simulink model "FaceDet_x4"  (Simulink 7.7)
settings: Solver=FixedStepDiscrete  StartTime=0  StopTime=10  RelTol=1e-3
libraries: simulink x257
(part 3 of 5)

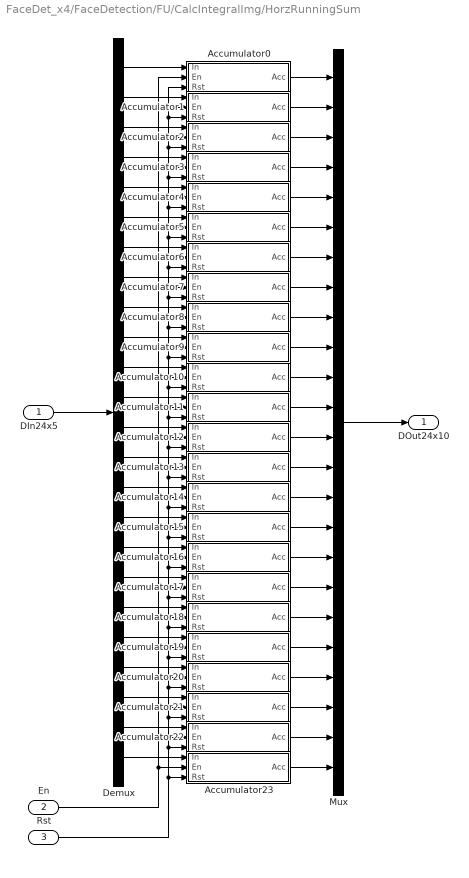
== system FaceDet_x4/FaceDetection/FU/CalcIntegralImg/HorzRunningSum ==
  DIn24x5 : Inport
  En : Inport  Port=2
  Rst : Inport  Port=3
  Accumulator0 : Subsystem  TreatAsAtomicUnit=on  mask(Accumulator){NBits=10}
      mask prompts: NBits "Number of Bits"
      mask help:
      | Accumulates incoming data. On reset only the state is initialized, meaning that when the reset is asserted the first valid output will be available from the next clock.
      | It is user responsiblity not to overcome the capacity of the accumulator.
      mask Help: web( ['E:\Ilia\Sightic\MakeVerilog\AccBlk\', 'AccBlkHelp.htm'] )
      mask Display: disp( 'Acc Blk\nBDelay = 0' )
  Accumulator1 : Subsystem  TreatAsAtomicUnit=on  mask(Accumulator){NBits=10}
      mask prompts: NBits "Number of Bits"
      mask help:
      | Accumulates incoming data. On reset only the state is initialized, meaning that when the reset is asserted the first valid output will be available from the next clock.
      | It is user responsiblity not to overcome the capacity of the accumulator.
      mask Help: web( ['E:\Ilia\Sightic\MakeVerilog\AccBlk\', 'AccBlkHelp.htm'] )
      mask Display: disp( 'Acc Blk\nBDelay = 0' )
  Accumulator10 : Subsystem  TreatAsAtomicUnit=on  mask(Accumulator){NBits=10}
      mask prompts: NBits "Number of Bits"
      mask help:
      | Accumulates incoming data. On reset only the state is initialized, meaning that when the reset is asserted the first valid output will be available from the next clock.
      | It is user responsiblity not to overcome the capacity of the accumulator.
      mask Help: web( ['E:\Ilia\Sightic\MakeVerilog\AccBlk\', 'AccBlkHelp.htm'] )
      mask Display: disp( 'Acc Blk\nBDelay = 0' )
  Accumulator11 : Subsystem  TreatAsAtomicUnit=on  mask(Accumulator){NBits=10}
      mask prompts: NBits "Number of Bits"
      mask help:
      | Accumulates incoming data. On reset only the state is initialized, meaning that when the reset is asserted the first valid output will be available from the next clock.
      | It is user responsiblity not to overcome the capacity of the accumulator.
      mask Help: web( ['E:\Ilia\Sightic\MakeVerilog\AccBlk\', 'AccBlkHelp.htm'] )
      mask Display: disp( 'Acc Blk\nBDelay = 0' )
  Accumulator12 : Subsystem  TreatAsAtomicUnit=on  mask(Accumulator){NBits=10}
      mask prompts: NBits "Number of Bits"
      mask help:
      | Accumulates incoming data. On reset only the state is initialized, meaning that when the reset is asserted the first valid output will be available from the next clock.
      | It is user responsiblity not to overcome the capacity of the accumulator.
      mask Help: web( ['E:\Ilia\Sightic\MakeVerilog\AccBlk\', 'AccBlkHelp.htm'] )
      mask Display: disp( 'Acc Blk\nBDelay = 0' )
  Accumulator13 : Subsystem  TreatAsAtomicUnit=on  mask(Accumulator){NBits=10}
      mask prompts: NBits "Number of Bits"
      mask help:
      | Accumulates incoming data. On reset only the state is initialized, meaning that when the reset is asserted the first valid output will be available from the next clock.
      | It is user responsiblity not to overcome the capacity of the accumulator.
      mask Help: web( ['E:\Ilia\Sightic\MakeVerilog\AccBlk\', 'AccBlkHelp.htm'] )
      mask Display: disp( 'Acc Blk\nBDelay = 0' )
  Accumulator14 : Subsystem  TreatAsAtomicUnit=on  mask(Accumulator){NBits=10}
      mask prompts: NBits "Number of Bits"
      mask help:
      | Accumulates incoming data. On reset only the state is initialized, meaning that when the reset is asserted the first valid output will be available from the next clock.
      | It is user responsiblity not to overcome the capacity of the accumulator.
      mask Help: web( ['E:\Ilia\Sightic\MakeVerilog\AccBlk\', 'AccBlkHelp.htm'] )
      mask Display: disp( 'Acc Blk\nBDelay = 0' )
  Accumulator15 : Subsystem  TreatAsAtomicUnit=on  mask(Accumulator){NBits=10}
      mask prompts: NBits "Number of Bits"
      mask help:
      | Accumulates incoming data. On reset only the state is initialized, meaning that when the reset is asserted the first valid output will be available from the next clock.
      | It is user responsiblity not to overcome the capacity of the accumulator.
      mask Help: web( ['E:\Ilia\Sightic\MakeVerilog\AccBlk\', 'AccBlkHelp.htm'] )
      mask Display: disp( 'Acc Blk\nBDelay = 0' )
  Accumulator16 : Subsystem  TreatAsAtomicUnit=on  mask(Accumulator){NBits=10}
      mask prompts: NBits "Number of Bits"
      mask help:
      | Accumulates incoming data. On reset only the state is initialized, meaning that when the reset is asserted the first valid output will be available from the next clock.
      | It is user responsiblity not to overcome the capacity of the accumulator.
      mask Help: web( ['E:\Ilia\Sightic\MakeVerilog\AccBlk\', 'AccBlkHelp.htm'] )
      mask Display: disp( 'Acc Blk\nBDelay = 0' )
  Accumulator17 : Subsystem  TreatAsAtomicUnit=on  mask(Accumulator){NBits=10}
      mask prompts: NBits "Number of Bits"
      mask help:
      | Accumulates incoming data. On reset only the state is initialized, meaning that when the reset is asserted the first valid output will be available from the next clock.
      | It is user responsiblity not to overcome the capacity of the accumulator.
      mask Help: web( ['E:\Ilia\Sightic\MakeVerilog\AccBlk\', 'AccBlkHelp.htm'] )
      mask Display: disp( 'Acc Blk\nBDelay = 0' )
  Accumulator18 : Subsystem  TreatAsAtomicUnit=on  mask(Accumulator){NBits=10}
      mask prompts: NBits "Number of Bits"
      mask help:
      | Accumulates incoming data. On reset only the state is initialized, meaning that when the reset is asserted the first valid output will be available from the next clock.
      | It is user responsiblity not to overcome the capacity of the accumulator.
      mask Help: web( ['E:\Ilia\Sightic\MakeVerilog\AccBlk\', 'AccBlkHelp.htm'] )
      mask Display: disp( 'Acc Blk\nBDelay = 0' )
  Accumulator19 : Subsystem  TreatAsAtomicUnit=on  mask(Accumulator){NBits=10}
      mask prompts: NBits "Number of Bits"
      mask help:
      | Accumulates incoming data. On reset only the state is initialized, meaning that when the reset is asserted the first valid output will be available from the next clock.
      | It is user responsiblity not to overcome the capacity of the accumulator.
      mask Help: web( ['E:\Ilia\Sightic\MakeVerilog\AccBlk\', 'AccBlkHelp.htm'] )
      mask Display: disp( 'Acc Blk\nBDelay = 0' )
  Accumulator2 : Subsystem  TreatAsAtomicUnit=on  mask(Accumulator){NBits=10}
      mask prompts: NBits "Number of Bits"
      mask help:
      | Accumulates incoming data. On reset only the state is initialized, meaning that when the reset is asserted the first valid output will be available from the next clock.
      | It is user responsiblity not to overcome the capacity of the accumulator.
      mask Help: web( ['E:\Ilia\Sightic\MakeVerilog\AccBlk\', 'AccBlkHelp.htm'] )
      mask Display: disp( 'Acc Blk\nBDelay = 0' )
  Accumulator20 : Subsystem  TreatAsAtomicUnit=on  mask(Accumulator){NBits=10}
      mask prompts: NBits "Number of Bits"
      mask help:
      | Accumulates incoming data. On reset only the state is initialized, meaning that when the reset is asserted the first valid output will be available from the next clock.
      | It is user responsiblity not to overcome the capacity of the accumulator.
      mask Help: web( ['E:\Ilia\Sightic\MakeVerilog\AccBlk\', 'AccBlkHelp.htm'] )
      mask Display: disp( 'Acc Blk\nBDelay = 0' )
  Accumulator21 : Subsystem  TreatAsAtomicUnit=on  mask(Accumulator){NBits=10}
      mask prompts: NBits "Number of Bits"
      mask help:
      | Accumulates incoming data. On reset only the state is initialized, meaning that when the reset is asserted the first valid output will be available from the next clock.
      | It is user responsiblity not to overcome the capacity of the accumulator.
      mask Help: web( ['E:\Ilia\Sightic\MakeVerilog\AccBlk\', 'AccBlkHelp.htm'] )
      mask Display: disp( 'Acc Blk\nBDelay = 0' )
  Accumulator22 : Subsystem  TreatAsAtomicUnit=on  mask(Accumulator){NBits=10}
      mask prompts: NBits "Number of Bits"
      mask help:
      | Accumulates incoming data. On reset only the state is initialized, meaning that when the reset is asserted the first valid output will be available from the next clock.
      | It is user responsiblity not to overcome the capacity of the accumulator.
      mask Help: web( ['E:\Ilia\Sightic\MakeVerilog\AccBlk\', 'AccBlkHelp.htm'] )
      mask Display: disp( 'Acc Blk\nBDelay = 0' )
  Accumulator23 : Subsystem  TreatAsAtomicUnit=on  mask(Accumulator){NBits=10}
      mask prompts: NBits "Number of Bits"
      mask help:
      | Accumulates incoming data. On reset only the state is initialized, meaning that when the reset is asserted the first valid output will be available from the next clock.
      | It is user responsiblity not to overcome the capacity of the accumulator.
      mask Help: web( ['E:\Ilia\Sightic\MakeVerilog\AccBlk\', 'AccBlkHelp.htm'] )
      mask Display: disp( 'Acc Blk\nBDelay = 0' )
  Accumulator3 : Subsystem  TreatAsAtomicUnit=on  mask(Accumulator){NBits=10}
      mask prompts: NBits "Number of Bits"
      mask help:
      | Accumulates incoming data. On reset only the state is initialized, meaning that when the reset is asserted the first valid output will be available from the next clock.
      | It is user responsiblity not to overcome the capacity of the accumulator.
      mask Help: web( ['E:\Ilia\Sightic\MakeVerilog\AccBlk\', 'AccBlkHelp.htm'] )
      mask Display: disp( 'Acc Blk\nBDelay = 0' )
  Accumulator4 : Subsystem  TreatAsAtomicUnit=on  mask(Accumulator){NBits=10}
      mask prompts: NBits "Number of Bits"
      mask help:
      | Accumulates incoming data. On reset only the state is initialized, meaning that when the reset is asserted the first valid output will be available from the next clock.
      | It is user responsiblity not to overcome the capacity of the accumulator.
      mask Help: web( ['E:\Ilia\Sightic\MakeVerilog\AccBlk\', 'AccBlkHelp.htm'] )
      mask Display: disp( 'Acc Blk\nBDelay = 0' )
  Accumulator5 : Subsystem  TreatAsAtomicUnit=on  mask(Accumulator){NBits=10}
      mask prompts: NBits "Number of Bits"
      mask help:
      | Accumulates incoming data. On reset only the state is initialized, meaning that when the reset is asserted the first valid output will be available from the next clock.
      | It is user responsiblity not to overcome the capacity of the accumulator.
      mask Help: web( ['E:\Ilia\Sightic\MakeVerilog\AccBlk\', 'AccBlkHelp.htm'] )
      mask Display: disp( 'Acc Blk\nBDelay = 0' )
  Accumulator6 : Subsystem  TreatAsAtomicUnit=on  mask(Accumulator){NBits=10}
      mask prompts: NBits "Number of Bits"
      mask help:
      | Accumulates incoming data. On reset only the state is initialized, meaning that when the reset is asserted the first valid output will be available from the next clock.
      | It is user responsiblity not to overcome the capacity of the accumulator.
      mask Help: web( ['E:\Ilia\Sightic\MakeVerilog\AccBlk\', 'AccBlkHelp.htm'] )
      mask Display: disp( 'Acc Blk\nBDelay = 0' )
  Accumulator7 : Subsystem  TreatAsAtomicUnit=on  mask(Accumulator){NBits=10}
      mask prompts: NBits "Number of Bits"
      mask help:
      | Accumulates incoming data. On reset only the state is initialized, meaning that when the reset is asserted the first valid output will be available from the next clock.
      | It is user responsiblity not to overcome the capacity of the accumulator.
      mask Help: web( ['E:\Ilia\Sightic\MakeVerilog\AccBlk\', 'AccBlkHelp.htm'] )
      mask Display: disp( 'Acc Blk\nBDelay = 0' )
  Accumulator8 : Subsystem  TreatAsAtomicUnit=on  mask(Accumulator){NBits=10}
      mask prompts: NBits "Number of Bits"
      mask help:
      | Accumulates incoming data. On reset only the state is initialized, meaning that when the reset is asserted the first valid output will be available from the next clock.
      | It is user responsiblity not to overcome the capacity of the accumulator.
      mask Help: web( ['E:\Ilia\Sightic\MakeVerilog\AccBlk\', 'AccBlkHelp.htm'] )
      mask Display: disp( 'Acc Blk\nBDelay = 0' )
  Accumulator9 : Subsystem  TreatAsAtomicUnit=on  mask(Accumulator){NBits=10}
      mask prompts: NBits "Number of Bits"
      mask help:
      | Accumulates incoming data. On reset only the state is initialized, meaning that when the reset is asserted the first valid output will be available from the next clock.
      | It is user responsiblity not to overcome the capacity of the accumulator.
      mask Help: web( ['E:\Ilia\Sightic\MakeVerilog\AccBlk\', 'AccBlkHelp.htm'] )
      mask Display: disp( 'Acc Blk\nBDelay = 0' )
  Demux : Demux  Outputs=24
  Mux : Mux  Inputs=24
  DOut24x10 : Outport  RequirementInfo={} %GIDa_f25d4dfd_08ec_4fe4_83ec_06833589800f
  wires:
  DIn24x5/1 -> Demux/1
  Mux/1 -> DOut24x10/1
  Demux/1 -> Accumulator0/1(In)
  Demux/2 -> Accumulator1/1(In)
  Demux/3 -> Accumulator2/1(In)
  Demux/4 -> Accumulator3/1(In)
  Demux/5 -> Accumulator4/1(In)
  Demux/6 -> Accumulator5/1(In)
  Demux/7 -> Accumulator6/1(In)
  Demux/8 -> Accumulator7/1(In)
  Demux/9 -> Accumulator8/1(In)
  Demux/10 -> Accumulator9/1(In)
  Demux/11 -> Accumulator10/1(In)
  Demux/12 -> Accumulator11/1(In)
  Demux/13 -> Accumulator12/1(In)
  Demux/14 -> Accumulator13/1(In)
  Demux/15 -> Accumulator14/1(In)
  Demux/16 -> Accumulator15/1(In)
  Demux/17 -> Accumulator16/1(In)
  Demux/18 -> Accumulator17/1(In)
  Demux/19 -> Accumulator18/1(In)
  Demux/20 -> Accumulator19/1(In)
  Demux/21 -> Accumulator20/1(In)
  Demux/22 -> Accumulator21/1(In)
  Demux/23 -> Accumulator22/1(In)
  Demux/24 -> Accumulator23/1(In)
  En/1 -> Accumulator0/2(En), Accumulator1/2(En), Accumulator2/2(En), Accumulator3/2(En), Accumulator4/2(En), Accumulator5/2(En), Accumulator6/2(En), Accumulator7/2(En), Accumulator8/2(En), Accumulator9/2(En), Accumulator10/2(En), Accumulator11/2(En), Accumulator12/2(En), Accumulator13/2(En), Accumulator14/2(En), Accumulator15/2(En), Accumulator16/2(En), Accumulator17/2(En), Accumulator18/2(En), Accumulator19/2(En), Accumulator20/2(En), Accumulator21/2(En), Accumulator22/2(En), Accumulator23/2(En)
  Rst/1 -> Accumulator0/3(Rst), Accumulator1/3(Rst), Accumulator2/3(Rst), Accumulator3/3(Rst), Accumulator4/3(Rst), Accumulator5/3(Rst), Accumulator6/3(Rst), Accumulator7/3(Rst), Accumulator8/3(Rst), Accumulator9/3(Rst), Accumulator10/3(Rst), Accumulator11/3(Rst), Accumulator12/3(Rst), Accumulator13/3(Rst), Accumulator14/3(Rst), Accumulator15/3(Rst), Accumulator16/3(Rst), Accumulator17/3(Rst), Accumulator18/3(Rst), Accumulator19/3(Rst), Accumulator20/3(Rst), Accumulator21/3(Rst), Accumulator22/3(Rst), Accumulator23/3(Rst)
  Accumulator0/1(Acc) -> Mux/1
  Accumulator1/1(Acc) -> Mux/2
  Accumulator2/1(Acc) -> Mux/3
  Accumulator3/1(Acc) -> Mux/4
  Accumulator4/1(Acc) -> Mux/5
  Accumulator5/1(Acc) -> Mux/6
  Accumulator6/1(Acc) -> Mux/7
  Accumulator7/1(Acc) -> Mux/8
  Accumulator8/1(Acc) -> Mux/9
  Accumulator9/1(Acc) -> Mux/10
  Accumulator10/1(Acc) -> Mux/11
  Accumulator11/1(Acc) -> Mux/12
  Accumulator12/1(Acc) -> Mux/13
  Accumulator13/1(Acc) -> Mux/14
  Accumulator14/1(Acc) -> Mux/15
  Accumulator15/1(Acc) -> Mux/16
  Accumulator16/1(Acc) -> Mux/17
  Accumulator17/1(Acc) -> Mux/18
  Accumulator18/1(Acc) -> Mux/19
  Accumulator19/1(Acc) -> Mux/20
  Accumulator20/1(Acc) -> Mux/21
  Accumulator21/1(Acc) -> Mux/22
  Accumulator22/1(Acc) -> Mux/23
  Accumulator23/1(Acc) -> Mux/24

== system FaceDet_x4/FaceDetection/FU/CalcIntegralImg/TestValidNN ==
  MeanBlkVal : Inport
  Logical Operator : Logic  Operator=OR  AllPortsSameDT=off  OutDataTypeStr=boolean
  MeanMax : Constant  Value=17508  OutDataTypeStr=ufix(15)
  MeanMin : Constant  Value=1543  OutDataTypeStr=ufix(11)
  PassFail : Logic  Operator=NOT  AllPortsSameDT=off  OutDataTypeStr=boolean
  UnitDelay : UnitDelay
  aboveMax : RelationalOperator  Operator=>  OutDataTypeStr=boolean
  belowMin : RelationalOperator  Operator=<  OutDataTypeStr=boolean
  ValidNN : Outport
  wires:
  MeanMin/1 -> belowMin/2
  MeanBlkVal/1 -> belowMin/1, aboveMax/1
  aboveMax/1 -> Logical Operator/1
  belowMin/1 -> Logical Operator/2
  Logical Operator/1 -> PassFail/1
  MeanMax/1 -> aboveMax/2
  PassFail/1 -> UnitDelay/1
  UnitDelay/1 -> ValidNN/1

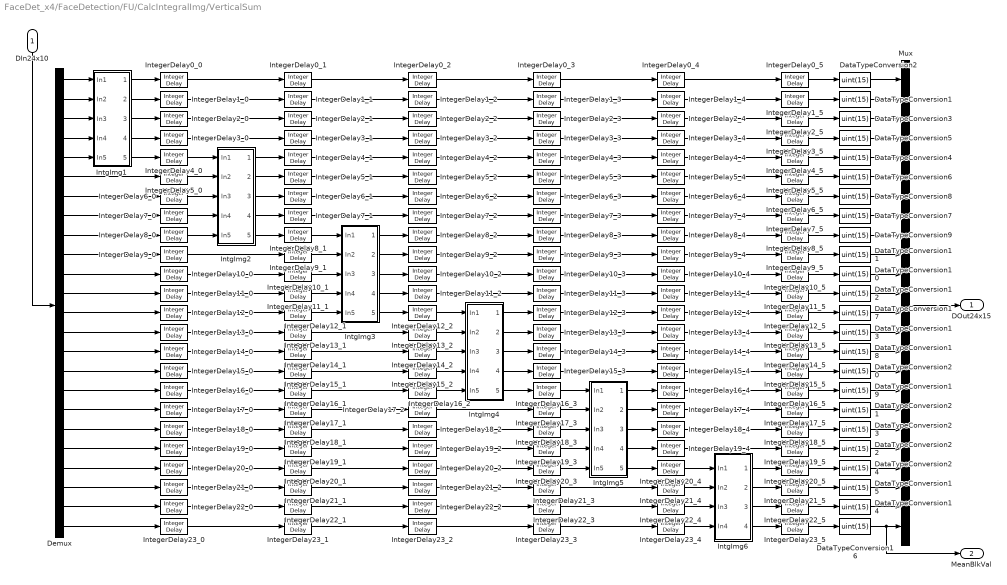
== system FaceDet_x4/FaceDetection/FU/CalcIntegralImg/VerticalSum ==
  DIn24x10 : Inport
  DataTypeConversion{1..24} (24 alike) : DataTypeConversion  OutDataTypeStr=uint(15)
  Demux : Demux  Outputs=24
  IntegerDelay0_{0..5} (6 alike) : simulink/Discrete/Integer Delay  NumDelays=1  InputProcessing=Inherited  vinit=0  samptime=1
  IntegerDelay10_{0..5} (6 alike) : simulink/Discrete/Integer Delay  NumDelays=1  InputProcessing=Inherited  vinit=0  samptime=1
  IntegerDelay11_{0..5} (6 alike) : simulink/Discrete/Integer Delay  NumDelays=1  InputProcessing=Inherited  vinit=0  samptime=1
  IntegerDelay12_{0..5} (6 alike) : simulink/Discrete/Integer Delay  NumDelays=1  InputProcessing=Inherited  vinit=0  samptime=1
  IntegerDelay13_{0..5} (6 alike) : simulink/Discrete/Integer Delay  NumDelays=1  InputProcessing=Inherited  vinit=0  samptime=1
  IntegerDelay14_{0..5} (6 alike) : simulink/Discrete/Integer Delay  NumDelays=1  InputProcessing=Inherited  vinit=0  samptime=1
  IntegerDelay15_{0..5} (6 alike) : simulink/Discrete/Integer Delay  NumDelays=1  InputProcessing=Inherited  vinit=0  samptime=1
  IntegerDelay16_{0..5} (6 alike) : simulink/Discrete/Integer Delay  NumDelays=1  InputProcessing=Inherited  vinit=0  samptime=1
  IntegerDelay17_{0..5} (6 alike) : simulink/Discrete/Integer Delay  NumDelays=1  InputProcessing=Inherited  vinit=0  samptime=1
  IntegerDelay18_{0..5} (6 alike) : simulink/Discrete/Integer Delay  NumDelays=1  InputProcessing=Inherited  vinit=0  samptime=1
  IntegerDelay19_{0..5} (6 alike) : simulink/Discrete/Integer Delay  NumDelays=1  InputProcessing=Inherited  vinit=0  samptime=1
  IntegerDelay1_{0..5} (6 alike) : simulink/Discrete/Integer Delay  NumDelays=1  InputProcessing=Inherited  vinit=0  samptime=1
  IntegerDelay20_{0..5} (6 alike) : simulink/Discrete/Integer Delay  NumDelays=1  InputProcessing=Inherited  vinit=0  samptime=1
  IntegerDelay21_{0..5} (6 alike) : simulink/Discrete/Integer Delay  NumDelays=1  InputProcessing=Inherited  vinit=0  samptime=1
  IntegerDelay22_{0..5} (6 alike) : simulink/Discrete/Integer Delay  NumDelays=1  InputProcessing=Inherited  vinit=0  samptime=1
  IntegerDelay23_{0..5} (6 alike) : simulink/Discrete/Integer Delay  NumDelays=1  InputProcessing=Inherited  vinit=0  samptime=1
  IntegerDelay2_{0..5} (6 alike) : simulink/Discrete/Integer Delay  NumDelays=1  InputProcessing=Inherited  vinit=0  samptime=1
  IntegerDelay3_{0..5} (6 alike) : simulink/Discrete/Integer Delay  NumDelays=1  InputProcessing=Inherited  vinit=0  samptime=1
  IntegerDelay4_{0..5} (6 alike) : simulink/Discrete/Integer Delay  NumDelays=1  InputProcessing=Inherited  vinit=0  samptime=1
  IntegerDelay5_{0..5} (6 alike) : simulink/Discrete/Integer Delay  NumDelays=1  InputProcessing=Inherited  vinit=0  samptime=1
  IntegerDelay6_{0..5} (6 alike) : simulink/Discrete/Integer Delay  NumDelays=1  InputProcessing=Inherited  vinit=0  samptime=1
  IntegerDelay7_{0..5} (6 alike) : simulink/Discrete/Integer Delay  NumDelays=1  InputProcessing=Inherited  vinit=0  samptime=1
  IntegerDelay8_{0..5} (6 alike) : simulink/Discrete/Integer Delay  NumDelays=1  InputProcessing=Inherited  vinit=0  samptime=1
  IntegerDelay9_{0..5} (6 alike) : simulink/Discrete/Integer Delay  NumDelays=1  InputProcessing=Inherited  vinit=0  samptime=1
  IntgImg1 : Subsystem
  IntgImg2 : Subsystem
  IntgImg3 : Subsystem
  IntgImg4 : Subsystem
  IntgImg5 : Subsystem
  IntgImg6 : Subsystem
  Mux : Mux  Inputs=24
  DOut24x15 : Outport
  MeanBlkVal : Outport  Port=2
  wires:
  DIn24x10/1 -> Demux/1
  Demux/1 -> IntgImg1/1(In1)
  Demux/2 -> IntgImg1/2(In2)
  Demux/3 -> IntgImg1/3(In3)
  Demux/6 -> IntegerDelay5_0/1
  IntgImg1/3(Out3) -> IntegerDelay2_0/1
  IntgImg1/1(Out1) -> IntegerDelay0_0/1
  Mux/1 -> DOut24x15/1
  IntgImg1/2(Out2) -> IntegerDelay1_0/1
  IntegerDelay2_0/1 -> IntegerDelay2_1/1
  IntegerDelay3_0/1 -> IntegerDelay3_1/1
  IntegerDelay4_0/1 -> IntgImg2/1(In1)
  Demux/7 -> IntegerDelay6_0/1
  IntegerDelay0_0/1 -> IntegerDelay0_1/1
  Demux/8 -> IntegerDelay7_0/1
  Demux/9 -> IntegerDelay8_0/1
  Demux/10 -> IntegerDelay9_0/1
  Demux/11 -> IntegerDelay10_0/1
  Demux/12 -> IntegerDelay11_0/1
  Demux/13 -> IntegerDelay12_0/1
  Demux/14 -> IntegerDelay13_0/1
  Demux/15 -> IntegerDelay14_0/1
  Demux/16 -> IntegerDelay15_0/1
  Demux/17 -> IntegerDelay16_0/1
  Demux/18 -> IntegerDelay17_0/1
  Demux/19 -> IntegerDelay18_0/1
  Demux/20 -> IntegerDelay19_0/1
  Demux/21 -> IntegerDelay20_0/1
  Demux/22 -> IntegerDelay21_0/1
  Demux/23 -> IntegerDelay22_0/1
  Demux/24 -> IntegerDelay23_0/1
  IntgImg2/1(Out1) -> IntegerDelay4_1/1
  IntegerDelay9_0/1 -> IntegerDelay9_1/1
  IntegerDelay10_0/1 -> IntegerDelay10_1/1
  IntegerDelay11_0/1 -> IntegerDelay11_1/1
  IntegerDelay12_0/1 -> IntegerDelay12_1/1
  IntegerDelay13_0/1 -> IntegerDelay13_1/1
  IntegerDelay14_0/1 -> IntegerDelay14_1/1
  IntegerDelay15_0/1 -> IntegerDelay15_1/1
  IntegerDelay16_0/1 -> IntegerDelay16_1/1
  IntegerDelay17_0/1 -> IntegerDelay17_1/1
  IntegerDelay18_0/1 -> IntegerDelay18_1/1
  IntegerDelay19_0/1 -> IntegerDelay19_1/1
  IntegerDelay20_0/1 -> IntegerDelay20_1/1
  IntegerDelay21_0/1 -> IntegerDelay21_1/1
  IntegerDelay22_0/1 -> IntegerDelay22_1/1
  IntegerDelay23_0/1 -> IntegerDelay23_1/1
  Demux/4 -> IntgImg1/4(In4)
  Demux/5 -> IntgImg1/5(In5)
  IntgImg1/4(Out4) -> IntegerDelay3_0/1
  IntgImg1/5(Out5) -> IntegerDelay4_0/1
  IntegerDelay1_0/1 -> IntegerDelay1_1/1
  IntegerDelay5_0/1 -> IntgImg2/2(In2)
  IntegerDelay6_0/1 -> IntgImg2/3(In3)
  IntegerDelay7_0/1 -> IntgImg2/4(In4)
  IntegerDelay8_0/1 -> IntgImg2/5(In5)
  IntgImg2/2(Out2) -> IntegerDelay5_1/1
  IntgImg2/3(Out3) -> IntegerDelay6_1/1
  IntgImg2/4(Out4) -> IntegerDelay7_1/1
  IntgImg2/5(Out5) -> IntegerDelay8_1/1
  IntegerDelay2_1/1 -> IntegerDelay2_2/1
  IntegerDelay3_1/1 -> IntegerDelay3_2/1
  IntegerDelay0_1/1 -> IntegerDelay0_2/1
  IntegerDelay13_1/1 -> IntegerDelay13_2/1
  IntegerDelay14_1/1 -> IntegerDelay14_2/1
  IntegerDelay15_1/1 -> IntegerDelay15_2/1
  IntegerDelay16_1/1 -> IntegerDelay16_2/1
  IntegerDelay17_1/1 -> IntegerDelay17_2/1
  IntegerDelay18_1/1 -> IntegerDelay18_2/1
  IntegerDelay19_1/1 -> IntegerDelay19_2/1
  IntegerDelay20_1/1 -> IntegerDelay20_2/1
  IntegerDelay21_1/1 -> IntegerDelay21_2/1
  IntegerDelay22_1/1 -> IntegerDelay22_2/1
  IntegerDelay23_1/1 -> IntegerDelay23_2/1
  IntegerDelay1_1/1 -> IntegerDelay1_2/1
  IntegerDelay8_1/1 -> IntgImg3/1(In1)
  IntegerDelay9_1/1 -> IntgImg3/2(In2)
  IntegerDelay10_1/1 -> IntgImg3/3(In3)
  IntegerDelay11_1/1 -> IntgImg3/4(In4)
  IntegerDelay12_1/1 -> IntgImg3/5(In5)
  IntegerDelay4_1/1 -> IntegerDelay4_2/1
  IntegerDelay5_1/1 -> IntegerDelay5_2/1
  IntegerDelay6_1/1 -> IntegerDelay6_2/1
  IntegerDelay7_1/1 -> IntegerDelay7_2/1
  IntgImg3/1(Out1) -> IntegerDelay8_2/1
  IntgImg3/2(Out2) -> IntegerDelay9_2/1
  IntgImg3/3(Out3) -> IntegerDelay10_2/1
  IntgImg3/4(Out4) -> IntegerDelay11_2/1
  IntgImg3/5(Out5) -> IntegerDelay12_2/1
  IntegerDelay2_2/1 -> IntegerDelay2_3/1
  IntegerDelay3_2/1 -> IntegerDelay3_3/1
  IntegerDelay0_2/1 -> IntegerDelay0_3/1
  IntegerDelay17_2/1 -> IntegerDelay17_3/1
  IntegerDelay18_2/1 -> IntegerDelay18_3/1
  IntegerDelay19_2/1 -> IntegerDelay19_3/1
  IntegerDelay20_2/1 -> IntegerDelay20_3/1
  IntegerDelay21_2/1 -> IntegerDelay21_3/1
  IntegerDelay22_2/1 -> IntegerDelay22_3/1
  IntegerDelay23_2/1 -> IntegerDelay23_3/1
  IntegerDelay1_2/1 -> IntegerDelay1_3/1
  IntegerDelay4_2/1 -> IntegerDelay4_3/1
  IntegerDelay5_2/1 -> IntegerDelay5_3/1
  IntegerDelay6_2/1 -> IntegerDelay6_3/1
  IntegerDelay7_2/1 -> IntegerDelay7_3/1
  IntegerDelay8_2/1 -> IntegerDelay8_3/1
  IntegerDelay9_2/1 -> IntegerDelay9_3/1
  IntegerDelay10_2/1 -> IntegerDelay10_3/1
  IntegerDelay11_2/1 -> IntegerDelay11_3/1
  IntegerDelay12_2/1 -> IntgImg4/1(In1)
  IntegerDelay13_2/1 -> IntgImg4/2(In2)
  IntegerDelay14_2/1 -> IntgImg4/3(In3)
  IntegerDelay15_2/1 -> IntgImg4/4(In4)
  IntegerDelay16_2/1 -> IntgImg4/5(In5)
  IntgImg4/1(Out1) -> IntegerDelay12_3/1
  IntgImg4/2(Out2) -> IntegerDelay13_3/1
  IntgImg4/3(Out3) -> IntegerDelay14_3/1
  IntgImg4/4(Out4) -> IntegerDelay15_3/1
  IntgImg4/5(Out5) -> IntegerDelay16_3/1
  IntegerDelay2_3/1 -> IntegerDelay2_4/1
  IntegerDelay3_3/1 -> IntegerDelay3_4/1
  IntegerDelay0_3/1 -> IntegerDelay0_4/1
  IntegerDelay21_3/1 -> IntegerDelay21_4/1
  IntegerDelay22_3/1 -> IntegerDelay22_4/1
  IntegerDelay23_3/1 -> IntegerDelay23_4/1
  IntegerDelay1_3/1 -> IntegerDelay1_4/1
  IntegerDelay4_3/1 -> IntegerDelay4_4/1
  IntegerDelay5_3/1 -> IntegerDelay5_4/1
  IntegerDelay6_3/1 -> IntegerDelay6_4/1
  IntegerDelay7_3/1 -> IntegerDelay7_4/1
  IntegerDelay8_3/1 -> IntegerDelay8_4/1
  IntegerDelay9_3/1 -> IntegerDelay9_4/1
  IntegerDelay10_3/1 -> IntegerDelay10_4/1
  IntegerDelay11_3/1 -> IntegerDelay11_4/1
  IntegerDelay12_3/1 -> IntegerDelay12_4/1
  IntegerDelay13_3/1 -> IntegerDelay13_4/1
  IntegerDelay14_3/1 -> IntegerDelay14_4/1
  IntegerDelay15_3/1 -> IntegerDelay15_4/1
  IntegerDelay16_3/1 -> IntgImg5/1(In1)
  IntegerDelay17_3/1 -> IntgImg5/2(In2)
  IntegerDelay18_3/1 -> IntgImg5/3(In3)
  IntegerDelay19_3/1 -> IntgImg5/4(In4)
  IntegerDelay20_3/1 -> IntgImg5/5(In5)
  IntgImg5/1(Out1) -> IntegerDelay16_4/1
  IntgImg5/2(Out2) -> IntegerDelay17_4/1
  IntgImg5/3(Out3) -> IntegerDelay18_4/1
  IntgImg5/4(Out4) -> IntegerDelay19_4/1
  IntgImg5/5(Out5) -> IntegerDelay20_4/1
  IntegerDelay2_4/1 -> IntegerDelay2_5/1
  IntegerDelay3_4/1 -> IntegerDelay3_5/1
  IntegerDelay0_4/1 -> IntegerDelay0_5/1
  IntegerDelay1_4/1 -> IntegerDelay1_5/1
  IntegerDelay4_4/1 -> IntegerDelay4_5/1
  IntegerDelay5_4/1 -> IntegerDelay5_5/1
  IntegerDelay6_4/1 -> IntegerDelay6_5/1
  IntegerDelay7_4/1 -> IntegerDelay7_5/1
  IntegerDelay8_4/1 -> IntegerDelay8_5/1
  IntegerDelay9_4/1 -> IntegerDelay9_5/1
  IntegerDelay10_4/1 -> IntegerDelay10_5/1
  IntegerDelay11_4/1 -> IntegerDelay11_5/1
  IntegerDelay12_4/1 -> IntegerDelay12_5/1
  IntegerDelay13_4/1 -> IntegerDelay13_5/1
  IntegerDelay14_4/1 -> IntegerDelay14_5/1
  IntegerDelay15_4/1 -> IntegerDelay15_5/1
  IntegerDelay16_4/1 -> IntegerDelay16_5/1
  IntegerDelay17_4/1 -> IntegerDelay17_5/1
  IntegerDelay18_4/1 -> IntegerDelay18_5/1
  IntegerDelay19_4/1 -> IntegerDelay19_5/1
  IntegerDelay20_4/1 -> IntgImg6/1(In1)
  IntegerDelay21_4/1 -> IntgImg6/2(In2)
  IntegerDelay22_4/1 -> IntgImg6/3(In3)
  IntegerDelay23_4/1 -> IntgImg6/4(In4)
  IntgImg6/1(Out1) -> IntegerDelay20_5/1
  IntgImg6/2(Out2) -> IntegerDelay21_5/1
  IntgImg6/3(Out3) -> IntegerDelay22_5/1
  IntgImg6/4(Out4) -> IntegerDelay23_5/1
  IntegerDelay0_5/1 -> DataTypeConversion2/1
  IntegerDelay1_5/1 -> DataTypeConversion1/1
  IntegerDelay2_5/1 -> DataTypeConversion3/1
  IntegerDelay3_5/1 -> DataTypeConversion5/1
  IntegerDelay4_5/1 -> DataTypeConversion4/1
  IntegerDelay5_5/1 -> DataTypeConversion6/1
  IntegerDelay6_5/1 -> DataTypeConversion8/1
  IntegerDelay7_5/1 -> DataTypeConversion7/1
  IntegerDelay8_5/1 -> DataTypeConversion9/1
  IntegerDelay9_5/1 -> DataTypeConversion11/1
  IntegerDelay10_5/1 -> DataTypeConversion10/1
  IntegerDelay11_5/1 -> DataTypeConversion12/1
  IntegerDelay12_5/1 -> DataTypeConversion17/1
  IntegerDelay13_5/1 -> DataTypeConversion13/1
  IntegerDelay14_5/1 -> DataTypeConversion18/1
  IntegerDelay15_5/1 -> DataTypeConversion20/1
  IntegerDelay16_5/1 -> DataTypeConversion19/1
  IntegerDelay17_5/1 -> DataTypeConversion21/1
  IntegerDelay19_5/1 -> DataTypeConversion22/1
  IntegerDelay18_5/1 -> DataTypeConversion23/1
  IntegerDelay20_5/1 -> DataTypeConversion24/1
  IntegerDelay21_5/1 -> DataTypeConversion15/1
  IntegerDelay22_5/1 -> DataTypeConversion14/1
  IntegerDelay23_5/1 -> DataTypeConversion16/1
  DataTypeConversion2/1 -> Mux/1
  DataTypeConversion1/1 -> Mux/2
  DataTypeConversion3/1 -> Mux/3
  DataTypeConversion5/1 -> Mux/4
  DataTypeConversion4/1 -> Mux/5
  DataTypeConversion6/1 -> Mux/6
  DataTypeConversion8/1 -> Mux/7
  DataTypeConversion7/1 -> Mux/8
  DataTypeConversion9/1 -> Mux/9
  DataTypeConversion11/1 -> Mux/10
  DataTypeConversion10/1 -> Mux/11
  DataTypeConversion12/1 -> Mux/12
  DataTypeConversion17/1 -> Mux/13
  DataTypeConversion13/1 -> Mux/14
  DataTypeConversion18/1 -> Mux/15
  DataTypeConversion20/1 -> Mux/16
  DataTypeConversion19/1 -> Mux/17
  DataTypeConversion21/1 -> Mux/18
  DataTypeConversion23/1 -> Mux/19
  DataTypeConversion22/1 -> Mux/20
  DataTypeConversion24/1 -> Mux/21
  DataTypeConversion15/1 -> Mux/22
  DataTypeConversion14/1 -> Mux/23
  DataTypeConversion16/1 -> Mux/24, MeanBlkVal/1

== system FaceDet_x4/FaceDetection/FU/CalcNNVariance/AccVar ==
  note: AccumulatorBlock
  In : Inport
  En : Inport  Port=2
  Rst : Inport  Port=3
  Adder : Sum  OutDataTypeStr=uint(NBits)
  UDlyER : Subsystem  mask(Unit Delay Enabled Resettable){vinit=0, tsamp=-1}
      mask prompts: vinit "Initial condition:"; tsamp "Sample time:"
      mask help:
      | Normally, the output is the signal u delayed by one sample period.
      | When the reset signal R is true, the state is always set equal to the initial condition parameter.  This reset action is vectorized and supports scalar expansion.
      | When the enable signal is false, the block is disabled, and the state and output values do not change except for resets.  The enable action is vectorized and supports scalar expansion.
      mask Display: dpoly(1,[1 0],'z')
  Acc : Outport
  wires:
  UDlyER/1(y) -> Adder/2
  Adder/1 -> Acc/1, UDlyER/1(u)
  In/1 -> Adder/1
  Rst/1 -> UDlyER/3(R)
  En/1 -> UDlyER/2(E)

== system FaceDet_x4/FaceDetection/FU/CalcNNVariance/CounterModulo2 ==
  note: AccumulatorBlock
  In : Inport
  En : Inport  Port=2
  Rst : Inport  Port=3
  Adder : Sum  OutDataTypeStr=uint(NBits)
  UDlyER : Subsystem  mask(Unit Delay Enabled Resettable){vinit=0, tsamp=-1}
      mask prompts: vinit "Initial condition:"; tsamp "Sample time:"
      mask help:
      | Normally, the output is the signal u delayed by one sample period.
      | When the reset signal R is true, the state is always set equal to the initial condition parameter.  This reset action is vectorized and supports scalar expansion.
      | When the enable signal is false, the block is disabled, and the state and output values do not change except for resets.  The enable action is vectorized and supports scalar expansion.
      mask Display: dpoly(1,[1 0],'z')
  Acc : Outport
  wires:
  En/1 -> UDlyER/2(E)
  Rst/1 -> UDlyER/3(R)
  In/1 -> Adder/1
  Adder/1 -> UDlyER/1(u), Acc/1
  UDlyER/1(y) -> Adder/2

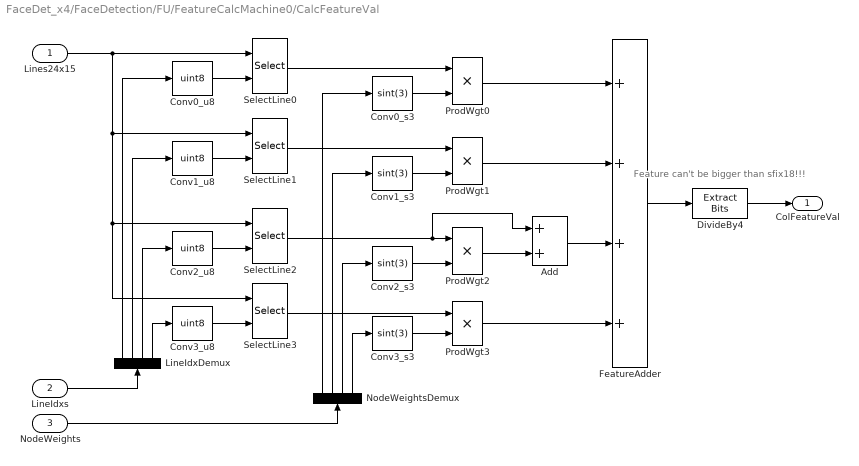
== system FaceDet_x4/FaceDetection/FU/FeatureCalcMachine0/CalcFeatureVal ==
  note: Feature can't be bigger
      | than sfix18!!!
  Lines24x15 : Inport
  LineIdxs : Inport  Port=2
  NodeWeights : Inport  Port=3
  Add : Sum  OutDataTypeStr=sint(18)
  Conv0_s3 : DataTypeConversion  OutDataTypeStr=sint(3)
  Conv0_u8 : DataTypeConversion  OutDataTypeStr=uint8
  Conv1_s3 : DataTypeConversion  OutDataTypeStr=sint(3)
  Conv1_u8 : DataTypeConversion  OutDataTypeStr=uint8
  Conv2_s3 : DataTypeConversion  OutDataTypeStr=sint(3)
  Conv2_u8 : DataTypeConversion  OutDataTypeStr=uint8
  Conv3_s3 : DataTypeConversion  OutDataTypeStr=sint(3)
  Conv3_u8 : DataTypeConversion  OutDataTypeStr=uint8
  DivideBy4 : simulink/Logic and Bit Operations/Extract Bits  SystemSampleTime=-1  bitsToExtract=Range of bits  numBits=8  bitIdxRange=[0 17]  outScalingMode=Treat bit field as an integer
  FeatureAdder : Sum  Inputs=++++  OutDataTypeStr=sint(20)
  LineIdxDemux : Demux
  NodeWeightsDemux : Demux
  ProdWgt{0..3} (4 alike) : Product  OutDataTypeStr=sint(18)  RndMeth=Zero
  SelectLine{0..3} (4 alike) : Selector  IndexMode=Zero-based  IndexOptions=Index vector (port)  Indices=1  OutputSizes=1
  ColFeatureVal : Outport
  wires:
  ProdWgt2/1 -> Add/2
  Conv2_s3/1 -> ProdWgt2/2
  Conv1_s3/1 -> ProdWgt1/2
  Conv0_s3/1 -> ProdWgt0/2
  DivideBy4/1 -> ColFeatureVal/1
  Conv3_s3/1 -> ProdWgt3/2
  NodeWeightsDemux/1 -> Conv0_s3/1
  NodeWeightsDemux/2 -> Conv1_s3/1
  NodeWeightsDemux/3 -> Conv2_s3/1
  NodeWeightsDemux/4 -> Conv3_s3/1
  NodeWeights/1 -> NodeWeightsDemux/1
  LineIdxDemux/3 -> Conv2_u8/1
  LineIdxs/1 -> LineIdxDemux/1
  Lines24x15/1 -> SelectLine0/1, SelectLine1/1, SelectLine3/1, SelectLine2/1
  SelectLine3/1 -> ProdWgt3/1
  Conv3_u8/1 -> SelectLine3/2
  LineIdxDemux/4 -> Conv3_u8/1
  SelectLine2/1 -> Add/1, ProdWgt2/1
  Conv2_u8/1 -> SelectLine2/2
  SelectLine1/1 -> ProdWgt1/1
  Conv1_u8/1 -> SelectLine1/2
  LineIdxDemux/2 -> Conv1_u8/1
  SelectLine0/1 -> ProdWgt0/1
  Conv0_u8/1 -> SelectLine0/2
  LineIdxDemux/1 -> Conv0_u8/1
  FeatureAdder/1 -> DivideBy4/1
  ProdWgt3/1 -> FeatureAdder/4
  Add/1 -> FeatureAdder/3
  ProdWgt1/1 -> FeatureAdder/2
  ProdWgt0/1 -> FeatureAdder/1

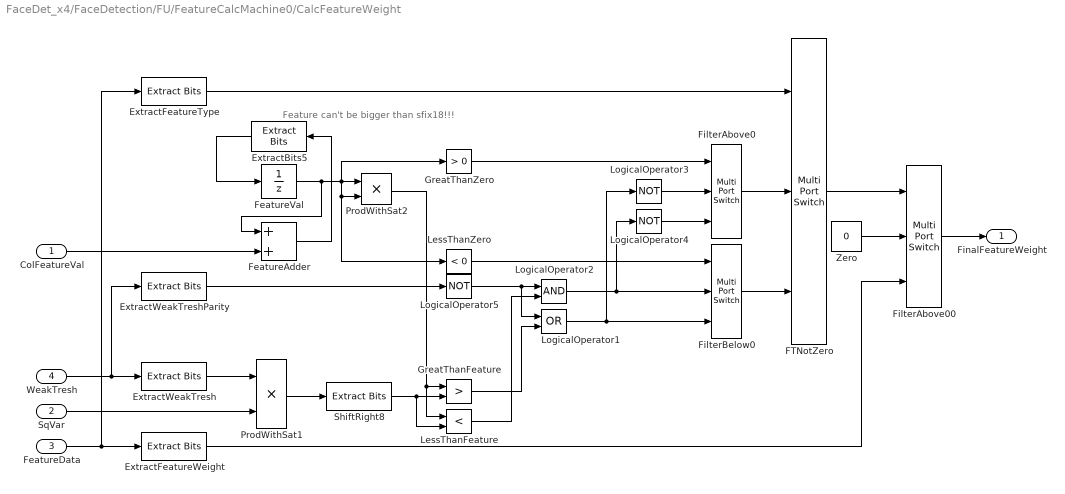
== system FaceDet_x4/FaceDetection/FU/FeatureCalcMachine0/CalcFeatureWeight ==
  note: Feature can't be bigger
      | than sfix18!!!
  ColFeatureVal : Inport
  SqVar : Inport  Port=2
  FeatureData : Inport  Port=3
  WeakTresh : Inport  Port=4
  ExtractBits5 : simulink/Logic and Bit Operations/Extract Bits  SystemSampleTime=-1  bitsToExtract=Range of bits  numBits=8  bitIdxRange=[0 17]  outScalingMode=Treat bit field as an integer
  ExtractFeatureType : simulink/Logic and Bit Operations/Extract Bits  SystemSampleTime=-1  bitsToExtract=Range of bits  numBits=8  bitIdxRange=[0 0]  outScalingMode=Treat bit field as an integer
  ExtractFeatureWeight : simulink/Logic and Bit Operations/Extract Bits  SystemSampleTime=-1  bitsToExtract=Range of bits  numBits=8  bitIdxRange=[1 16]  outScalingMode=Treat bit field as an integer
  ExtractWeakTresh : simulink/Logic and Bit Operations/Extract Bits  SystemSampleTime=-1  bitsToExtract=Range of bits  numBits=8  bitIdxRange=[1 24]  outScalingMode=Treat bit field as an integer
  ExtractWeakTreshParity : simulink/Logic and Bit Operations/Extract Bits  SystemSampleTime=-1  bitsToExtract=Range of bits  numBits=8  bitIdxRange=[0 0]  outScalingMode=Treat bit field as an integer
  FTNotZero : MultiPortSwitch  DataPortOrder=Zero-based contiguous  Inputs=2  zeroidx=on
  FeatureAdder : Sum  OutDataTypeStr=sint(19)
  FeatureVal : UnitDelay
  FilterAbove0 : MultiPortSwitch  DataPortOrder=Zero-based contiguous  Inputs=2  zeroidx=on
  FilterAbove00 : MultiPortSwitch  DataPortOrder=Zero-based contiguous  Inputs=2  zeroidx=on
  FilterBelow0 : MultiPortSwitch  DataPortOrder=Zero-based contiguous  Inputs=2  zeroidx=on
  GreatThanFeature : RelationalOperator  Operator=>  OutDataTypeStr=boolean
  GreatThanZero : simulink/Logic and Bit Operations/Compare To Zero  SystemSampleTime=-1  relop=>  LogicOutDataTypeMode=boolean  ZeroCross=off
  LessThanFeature : RelationalOperator  Operator=<  OutDataTypeStr=boolean
  LessThanZero : simulink/Logic and Bit Operations/Compare To Zero  SystemSampleTime=-1  relop=<  LogicOutDataTypeMode=boolean  ZeroCross=off
  LogicalOperator1 : Logic  Operator=OR  AllPortsSameDT=off  OutDataTypeStr=boolean
  LogicalOperator2 : Logic  AllPortsSameDT=off  OutDataTypeStr=boolean
  LogicalOperator3 : Logic  Operator=NOT  AllPortsSameDT=off  OutDataTypeStr=boolean
  LogicalOperator4 : Logic  Operator=NOT  AllPortsSameDT=off  OutDataTypeStr=boolean
  LogicalOperator5 : Logic  Operator=NOT  AllPortsSameDT=off  OutDataTypeStr=boolean
  ProdWithSat1 : Product  OutDataTypeStr=uint(32)  SaturateOnIntegerOverflow=on  RndMeth=Zero
  ProdWithSat2 : Product  OutDataTypeStr=uint32  SaturateOnIntegerOverflow=on  RndMeth=Zero
  ShiftRight8 : simulink/Logic and Bit Operations/Extract Bits  SystemSampleTime=-1  bitsToExtract=Range of bits  numBits=8  bitIdxRange=[8 31]  outScalingMode=Treat bit field as an integer
  Zero : Constant  Value=0  OutDataTypeStr=uint16
  FinalFeatureWeight : Outport
  wires:
  ExtractWeakTreshParity/1 -> LogicalOperator5/1
  ExtractWeakTresh/1 -> ProdWithSat1/1
  ExtractFeatureType/1 -> FTNotZero/1
  ExtractFeatureWeight/1 -> FilterAbove00/3
  ExtractBits5/1 -> FeatureVal/1
  ColFeatureVal/1 -> FeatureAdder/2
  FilterAbove00/1 -> FinalFeatureWeight/1
  FeatureData/1 -> ExtractFeatureType/1, ExtractFeatureWeight/1
  SqVar/1 -> ProdWithSat1/2
  WeakTresh/1 -> ExtractWeakTreshParity/1, ExtractWeakTresh/1
  GreatThanFeature/1 -> LogicalOperator1/2
  LogicalOperator1/1 -> FilterBelow0/3, LogicalOperator3/1
  LogicalOperator2/1 -> FilterBelow0/2, LogicalOperator4/1
  LessThanFeature/1 -> LogicalOperator2/2
  LogicalOperator5/1 -> LogicalOperator1/1, LogicalOperator2/1
  FTNotZero/1 -> FilterAbove00/1
  Zero/1 -> FilterAbove00/2
  LessThanZero/1 -> FilterBelow0/1
  GreatThanZero/1 -> FilterAbove0/1
  LogicalOperator3/1 -> FilterAbove0/2
  FilterAbove0/1 -> FTNotZero/2
  FilterBelow0/1 -> FTNotZero/3
  ProdWithSat1/1 -> ShiftRight8/1
  ShiftRight8/1 -> GreatThanFeature/2, LessThanFeature/2
  LogicalOperator4/1 -> FilterAbove0/3
  ProdWithSat2/1 -> LessThanFeature/1, GreatThanFeature/1
  FeatureAdder/1 -> ExtractBits5/1
  FeatureVal/1 -> ProdWithSat2/2, LessThanZero/1, ProdWithSat2/1, GreatThanZero/1, FeatureAdder/1

== system FaceDet_x4/FaceDetection/FU/FeatureCalcMachine1/CalcFeatureVal ==
  note: Feature can't be bigger
      | than sfix18!!!
  Lines24x15 : Inport
  LineIdxs : Inport  Port=2
  NodeWeights : Inport  Port=3
  Add : Sum  OutDataTypeStr=sint(18)
  Conv0_s3 : DataTypeConversion  OutDataTypeStr=sint(3)
  Conv0_u8 : DataTypeConversion  OutDataTypeStr=uint8
  Conv1_s3 : DataTypeConversion  OutDataTypeStr=sint(3)
  Conv1_u8 : DataTypeConversion  OutDataTypeStr=uint8
  Conv2_s3 : DataTypeConversion  OutDataTypeStr=sint(3)
  Conv2_u8 : DataTypeConversion  OutDataTypeStr=uint8
  Conv3_s3 : DataTypeConversion  OutDataTypeStr=sint(3)
  Conv3_u8 : DataTypeConversion  OutDataTypeStr=uint8
  DivideBy4 : simulink/Logic and Bit Operations/Extract Bits  SystemSampleTime=-1  bitsToExtract=Range of bits  numBits=8  bitIdxRange=[0 17]  outScalingMode=Treat bit field as an integer
  FeatureAdder : Sum  Inputs=++++  OutDataTypeStr=sint(20)
  LineIdxDemux : Demux
  NodeWeightsDemux : Demux
  ProdWgt{0..3} (4 alike) : Product  OutDataTypeStr=sint(18)  RndMeth=Zero
  SelectLine{0..3} (4 alike) : Selector  IndexMode=Zero-based  IndexOptions=Index vector (port)  Indices=1  OutputSizes=1
  ColFeatureVal : Outport
  wires:
  ProdWgt0/1 -> FeatureAdder/1
  ProdWgt1/1 -> FeatureAdder/2
  Add/1 -> FeatureAdder/3
  ProdWgt3/1 -> FeatureAdder/4
  FeatureAdder/1 -> DivideBy4/1
  LineIdxDemux/1 -> Conv0_u8/1
  Conv0_u8/1 -> SelectLine0/2
  SelectLine0/1 -> ProdWgt0/1
  LineIdxDemux/2 -> Conv1_u8/1
  Conv1_u8/1 -> SelectLine1/2
  SelectLine1/1 -> ProdWgt1/1
  Conv2_u8/1 -> SelectLine2/2
  SelectLine2/1 -> ProdWgt2/1, Add/1
  LineIdxDemux/4 -> Conv3_u8/1
  Conv3_u8/1 -> SelectLine3/2
  SelectLine3/1 -> ProdWgt3/1
  Lines24x15/1 -> SelectLine2/1, SelectLine3/1, SelectLine1/1, SelectLine0/1
  LineIdxs/1 -> LineIdxDemux/1
  LineIdxDemux/3 -> Conv2_u8/1
  NodeWeights/1 -> NodeWeightsDemux/1
  NodeWeightsDemux/4 -> Conv3_s3/1
  NodeWeightsDemux/3 -> Conv2_s3/1
  NodeWeightsDemux/2 -> Conv1_s3/1
  NodeWeightsDemux/1 -> Conv0_s3/1
  Conv3_s3/1 -> ProdWgt3/2
  DivideBy4/1 -> ColFeatureVal/1
  Conv0_s3/1 -> ProdWgt0/2
  Conv1_s3/1 -> ProdWgt1/2
  Conv2_s3/1 -> ProdWgt2/2
  ProdWgt2/1 -> Add/2

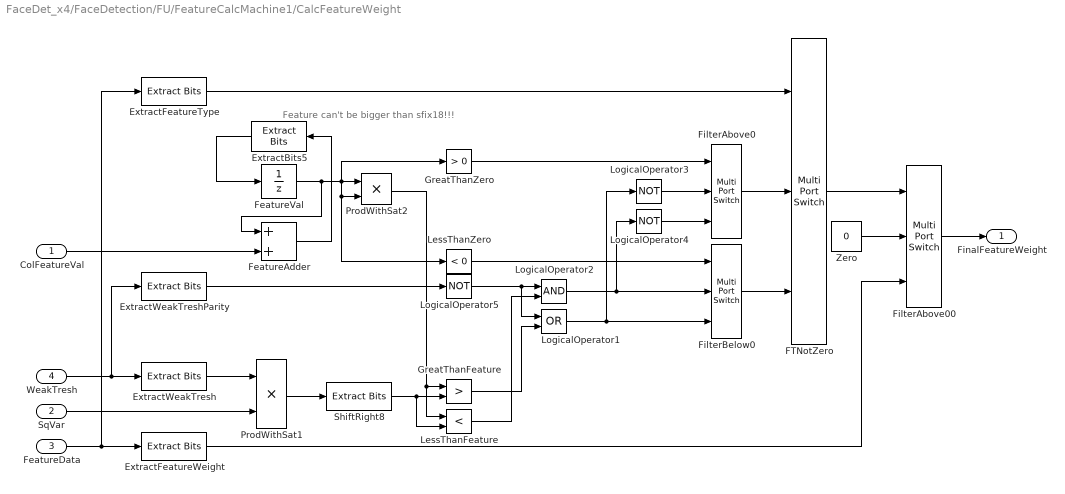
== system FaceDet_x4/FaceDetection/FU/FeatureCalcMachine1/CalcFeatureWeight ==
  note: Feature can't be bigger
      | than sfix18!!!
  ColFeatureVal : Inport
  SqVar : Inport  Port=2
  FeatureData : Inport  Port=3
  WeakTresh : Inport  Port=4
  ExtractBits5 : simulink/Logic and Bit Operations/Extract Bits  SystemSampleTime=-1  bitsToExtract=Range of bits  numBits=8  bitIdxRange=[0 17]  outScalingMode=Treat bit field as an integer
  ExtractFeatureType : simulink/Logic and Bit Operations/Extract Bits  SystemSampleTime=-1  bitsToExtract=Range of bits  numBits=8  bitIdxRange=[0 0]  outScalingMode=Treat bit field as an integer
  ExtractFeatureWeight : simulink/Logic and Bit Operations/Extract Bits  SystemSampleTime=-1  bitsToExtract=Range of bits  numBits=8  bitIdxRange=[1 16]  outScalingMode=Treat bit field as an integer
  ExtractWeakTresh : simulink/Logic and Bit Operations/Extract Bits  SystemSampleTime=-1  bitsToExtract=Range of bits  numBits=8  bitIdxRange=[1 24]  outScalingMode=Treat bit field as an integer
  ExtractWeakTreshParity : simulink/Logic and Bit Operations/Extract Bits  SystemSampleTime=-1  bitsToExtract=Range of bits  numBits=8  bitIdxRange=[0 0]  outScalingMode=Treat bit field as an integer
  FTNotZero : MultiPortSwitch  DataPortOrder=Zero-based contiguous  Inputs=2  zeroidx=on
  FeatureAdder : Sum  OutDataTypeStr=sint(19)
  FeatureVal : UnitDelay
  FilterAbove0 : MultiPortSwitch  DataPortOrder=Zero-based contiguous  Inputs=2  zeroidx=on
  FilterAbove00 : MultiPortSwitch  DataPortOrder=Zero-based contiguous  Inputs=2  zeroidx=on
  FilterBelow0 : MultiPortSwitch  DataPortOrder=Zero-based contiguous  Inputs=2  zeroidx=on
  GreatThanFeature : RelationalOperator  Operator=>  OutDataTypeStr=boolean
  GreatThanZero : simulink/Logic and Bit Operations/Compare To Zero  SystemSampleTime=-1  relop=>  LogicOutDataTypeMode=boolean  ZeroCross=off
  LessThanFeature : RelationalOperator  Operator=<  OutDataTypeStr=boolean
  LessThanZero : simulink/Logic and Bit Operations/Compare To Zero  SystemSampleTime=-1  relop=<  LogicOutDataTypeMode=boolean  ZeroCross=off
  LogicalOperator1 : Logic  Operator=OR  AllPortsSameDT=off  OutDataTypeStr=boolean
  LogicalOperator2 : Logic  AllPortsSameDT=off  OutDataTypeStr=boolean
  LogicalOperator3 : Logic  Operator=NOT  AllPortsSameDT=off  OutDataTypeStr=boolean
  LogicalOperator4 : Logic  Operator=NOT  AllPortsSameDT=off  OutDataTypeStr=boolean
  LogicalOperator5 : Logic  Operator=NOT  AllPortsSameDT=off  OutDataTypeStr=boolean
  ProdWithSat1 : Product  OutDataTypeStr=uint(32)  SaturateOnIntegerOverflow=on  RndMeth=Zero
  ProdWithSat2 : Product  OutDataTypeStr=uint32  SaturateOnIntegerOverflow=on  RndMeth=Zero
  ShiftRight8 : simulink/Logic and Bit Operations/Extract Bits  SystemSampleTime=-1  bitsToExtract=Range of bits  numBits=8  bitIdxRange=[8 31]  outScalingMode=Treat bit field as an integer
  Zero : Constant  Value=0  OutDataTypeStr=uint16
  FinalFeatureWeight : Outport
  wires:
  FeatureVal/1 -> FeatureAdder/1, GreatThanZero/1, ProdWithSat2/1, LessThanZero/1, ProdWithSat2/2
  FeatureAdder/1 -> ExtractBits5/1
  ProdWithSat2/1 -> GreatThanFeature/1, LessThanFeature/1
  LogicalOperator4/1 -> FilterAbove0/3
  ShiftRight8/1 -> LessThanFeature/2, GreatThanFeature/2
  ProdWithSat1/1 -> ShiftRight8/1
  FilterBelow0/1 -> FTNotZero/3
  FilterAbove0/1 -> FTNotZero/2
  LogicalOperator3/1 -> FilterAbove0/2
  GreatThanZero/1 -> FilterAbove0/1
  LessThanZero/1 -> FilterBelow0/1
  Zero/1 -> FilterAbove00/2
  FTNotZero/1 -> FilterAbove00/1
  LogicalOperator5/1 -> LogicalOperator2/1, LogicalOperator1/1
  LessThanFeature/1 -> LogicalOperator2/2
  LogicalOperator2/1 -> LogicalOperator4/1, FilterBelow0/2
  LogicalOperator1/1 -> LogicalOperator3/1, FilterBelow0/3
  GreatThanFeature/1 -> LogicalOperator1/2
  WeakTresh/1 -> ExtractWeakTresh/1, ExtractWeakTreshParity/1
  SqVar/1 -> ProdWithSat1/2
  FeatureData/1 -> ExtractFeatureWeight/1, ExtractFeatureType/1
  FilterAbove00/1 -> FinalFeatureWeight/1
  ColFeatureVal/1 -> FeatureAdder/2
  ExtractBits5/1 -> FeatureVal/1
  ExtractFeatureWeight/1 -> FilterAbove00/3
  ExtractFeatureType/1 -> FTNotZero/1
  ExtractWeakTresh/1 -> ProdWithSat1/1
  ExtractWeakTreshParity/1 -> LogicalOperator5/1

== system FaceDet_x4/FaceDetection/FU/FeatureCalcMachine2/CalcFeatureVal ==
  note: Feature can't be bigger
      | than sfix18!!!
  Lines24x15 : Inport
  LineIdxs : Inport  Port=2
  NodeWeights : Inport  Port=3
  Add : Sum  OutDataTypeStr=sint(18)
  Conv0_s3 : DataTypeConversion  OutDataTypeStr=sint(3)
  Conv0_u8 : DataTypeConversion  OutDataTypeStr=uint8
  Conv1_s3 : DataTypeConversion  OutDataTypeStr=sint(3)
  Conv1_u8 : DataTypeConversion  OutDataTypeStr=uint8
  Conv2_s3 : DataTypeConversion  OutDataTypeStr=sint(3)
  Conv2_u8 : DataTypeConversion  OutDataTypeStr=uint8
  Conv3_s3 : DataTypeConversion  OutDataTypeStr=sint(3)
  Conv3_u8 : DataTypeConversion  OutDataTypeStr=uint8
  DivideBy4 : simulink/Logic and Bit Operations/Extract Bits  SystemSampleTime=-1  bitsToExtract=Range of bits  numBits=8  bitIdxRange=[0 17]  outScalingMode=Treat bit field as an integer
  FeatureAdder : Sum  Inputs=++++  OutDataTypeStr=sint(20)
  LineIdxDemux : Demux
  NodeWeightsDemux : Demux
  ProdWgt{0..3} (4 alike) : Product  OutDataTypeStr=sint(18)  RndMeth=Zero
  SelectLine{0..3} (4 alike) : Selector  IndexMode=Zero-based  IndexOptions=Index vector (port)  Indices=1  OutputSizes=1
  ColFeatureVal : Outport
  wires:
  ProdWgt2/1 -> Add/2
  Conv2_s3/1 -> ProdWgt2/2
  Conv1_s3/1 -> ProdWgt1/2
  Conv0_s3/1 -> ProdWgt0/2
  DivideBy4/1 -> ColFeatureVal/1
  Conv3_s3/1 -> ProdWgt3/2
  NodeWeightsDemux/1 -> Conv0_s3/1
  NodeWeightsDemux/2 -> Conv1_s3/1
  NodeWeightsDemux/3 -> Conv2_s3/1
  NodeWeightsDemux/4 -> Conv3_s3/1
  NodeWeights/1 -> NodeWeightsDemux/1
  LineIdxDemux/3 -> Conv2_u8/1
  LineIdxs/1 -> LineIdxDemux/1
  Lines24x15/1 -> SelectLine0/1, SelectLine1/1, SelectLine3/1, SelectLine2/1
  SelectLine3/1 -> ProdWgt3/1
  Conv3_u8/1 -> SelectLine3/2
  LineIdxDemux/4 -> Conv3_u8/1
  SelectLine2/1 -> Add/1, ProdWgt2/1
  Conv2_u8/1 -> SelectLine2/2
  SelectLine1/1 -> ProdWgt1/1
  Conv1_u8/1 -> SelectLine1/2
  LineIdxDemux/2 -> Conv1_u8/1
  SelectLine0/1 -> ProdWgt0/1
  Conv0_u8/1 -> SelectLine0/2
  LineIdxDemux/1 -> Conv0_u8/1
  FeatureAdder/1 -> DivideBy4/1
  ProdWgt3/1 -> FeatureAdder/4
  Add/1 -> FeatureAdder/3
  ProdWgt1/1 -> FeatureAdder/2
  ProdWgt0/1 -> FeatureAdder/1

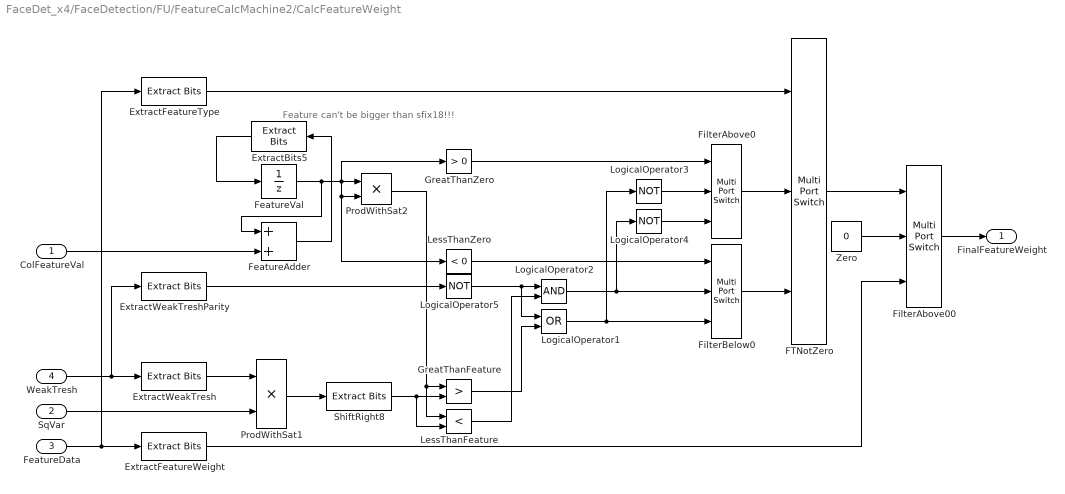
== system FaceDet_x4/FaceDetection/FU/FeatureCalcMachine2/CalcFeatureWeight ==
  note: Feature can't be bigger
      | than sfix18!!!
  ColFeatureVal : Inport
  SqVar : Inport  Port=2
  FeatureData : Inport  Port=3
  WeakTresh : Inport  Port=4
  ExtractBits5 : simulink/Logic and Bit Operations/Extract Bits  SystemSampleTime=-1  bitsToExtract=Range of bits  numBits=8  bitIdxRange=[0 17]  outScalingMode=Treat bit field as an integer
  ExtractFeatureType : simulink/Logic and Bit Operations/Extract Bits  SystemSampleTime=-1  bitsToExtract=Range of bits  numBits=8  bitIdxRange=[0 0]  outScalingMode=Treat bit field as an integer
  ExtractFeatureWeight : simulink/Logic and Bit Operations/Extract Bits  SystemSampleTime=-1  bitsToExtract=Range of bits  numBits=8  bitIdxRange=[1 16]  outScalingMode=Treat bit field as an integer
  ExtractWeakTresh : simulink/Logic and Bit Operations/Extract Bits  SystemSampleTime=-1  bitsToExtract=Range of bits  numBits=8  bitIdxRange=[1 24]  outScalingMode=Treat bit field as an integer
  ExtractWeakTreshParity : simulink/Logic and Bit Operations/Extract Bits  SystemSampleTime=-1  bitsToExtract=Range of bits  numBits=8  bitIdxRange=[0 0]  outScalingMode=Treat bit field as an integer
  FTNotZero : MultiPortSwitch  DataPortOrder=Zero-based contiguous  Inputs=2  zeroidx=on
  FeatureAdder : Sum  OutDataTypeStr=sint(19)
  FeatureVal : UnitDelay
  FilterAbove0 : MultiPortSwitch  DataPortOrder=Zero-based contiguous  Inputs=2  zeroidx=on
  FilterAbove00 : MultiPortSwitch  DataPortOrder=Zero-based contiguous  Inputs=2  zeroidx=on
  FilterBelow0 : MultiPortSwitch  DataPortOrder=Zero-based contiguous  Inputs=2  zeroidx=on
  GreatThanFeature : RelationalOperator  Operator=>  OutDataTypeStr=boolean
  GreatThanZero : simulink/Logic and Bit Operations/Compare To Zero  SystemSampleTime=-1  relop=>  LogicOutDataTypeMode=boolean  ZeroCross=off
  LessThanFeature : RelationalOperator  Operator=<  OutDataTypeStr=boolean
  LessThanZero : simulink/Logic and Bit Operations/Compare To Zero  SystemSampleTime=-1  relop=<  LogicOutDataTypeMode=boolean  ZeroCross=off
  LogicalOperator1 : Logic  Operator=OR  AllPortsSameDT=off  OutDataTypeStr=boolean
  LogicalOperator2 : Logic  AllPortsSameDT=off  OutDataTypeStr=boolean
  LogicalOperator3 : Logic  Operator=NOT  AllPortsSameDT=off  OutDataTypeStr=boolean
  LogicalOperator4 : Logic  Operator=NOT  AllPortsSameDT=off  OutDataTypeStr=boolean
  LogicalOperator5 : Logic  Operator=NOT  AllPortsSameDT=off  OutDataTypeStr=boolean
  ProdWithSat1 : Product  OutDataTypeStr=uint(32)  SaturateOnIntegerOverflow=on  RndMeth=Zero
  ProdWithSat2 : Product  OutDataTypeStr=uint32  SaturateOnIntegerOverflow=on  RndMeth=Zero
  ShiftRight8 : simulink/Logic and Bit Operations/Extract Bits  SystemSampleTime=-1  bitsToExtract=Range of bits  numBits=8  bitIdxRange=[8 31]  outScalingMode=Treat bit field as an integer
  Zero : Constant  Value=0  OutDataTypeStr=uint16
  FinalFeatureWeight : Outport
  wires:
  ExtractWeakTreshParity/1 -> LogicalOperator5/1
  ExtractWeakTresh/1 -> ProdWithSat1/1
  ExtractFeatureType/1 -> FTNotZero/1
  ExtractFeatureWeight/1 -> FilterAbove00/3
  ExtractBits5/1 -> FeatureVal/1
  ColFeatureVal/1 -> FeatureAdder/2
  FilterAbove00/1 -> FinalFeatureWeight/1
  FeatureData/1 -> ExtractFeatureType/1, ExtractFeatureWeight/1
  SqVar/1 -> ProdWithSat1/2
  WeakTresh/1 -> ExtractWeakTreshParity/1, ExtractWeakTresh/1
  GreatThanFeature/1 -> LogicalOperator1/2
  LogicalOperator1/1 -> FilterBelow0/3, LogicalOperator3/1
  LogicalOperator2/1 -> FilterBelow0/2, LogicalOperator4/1
  LessThanFeature/1 -> LogicalOperator2/2
  LogicalOperator5/1 -> LogicalOperator1/1, LogicalOperator2/1
  FTNotZero/1 -> FilterAbove00/1
  Zero/1 -> FilterAbove00/2
  LessThanZero/1 -> FilterBelow0/1
  GreatThanZero/1 -> FilterAbove0/1
  LogicalOperator3/1 -> FilterAbove0/2
  FilterAbove0/1 -> FTNotZero/2
  FilterBelow0/1 -> FTNotZero/3
  ProdWithSat1/1 -> ShiftRight8/1
  ShiftRight8/1 -> GreatThanFeature/2, LessThanFeature/2
  LogicalOperator4/1 -> FilterAbove0/3
  ProdWithSat2/1 -> LessThanFeature/1, GreatThanFeature/1
  FeatureAdder/1 -> ExtractBits5/1
  FeatureVal/1 -> ProdWithSat2/2, LessThanZero/1, ProdWithSat2/1, GreatThanZero/1, FeatureAdder/1
